simulink model "acc_and_enc"  (R2020a)
settings: Solver=FixedStepDiscrete  StartTime=0.0  StopTime=inf  FixedStep=.001  RelTol=1e-3  EnableMultiTasking=on
undefined symbols (not defined in the file): CAN_Device, Vector
libraries: sldrtlib x2
settings Model: SimulationMode=external  ExtModeTrigDuration=120000  ExtModeLogAll=off  Creator=quinteha  LastModifiedBy=rhyme
settings DataIOCC: LimitDataPoints=on  SaveFormat=Array  ReturnWorkspaceOutputs=off
settings OptimizationCC: ExpressionDepthLimit=2147483647
settings DebuggingCC: UnderspecifiedInitializationDetection=Classic  MergeDetectMultiDrivingBlocksExec=none  SolverPrmCheckMsg=warning  FcnCallInpInsideContextMsg=warning  StateNameClashWarn=warning  SFUnexpectedBacktrackingDiag=warning  SFNoUnconditionalDefaultTransitionDiag=warning  SFExecutionAtInitializationDiag=none  ArithmeticOperatorsInVariantConditions=warning
settings ModelReferenceCC: PropagateSignalLabelsOutOfModel=off
settings SFSimCC: SimUseLocalCustomCode=off  CustomCodeUndefinedFunction=UseInterfaceOnly
settings RTWCC: Description=Simulink Desktop Real-Time  SystemTargetFile=sldrt.tlc  TemplateMakefile=sldrt.tmf  RTWUseLocalCustomCode=off  RTWCompilerOptimization=on
settings CodeAppCC: MaxIdLength=95  StateflowObjectComments=on
settings SimulinkDesktopRealTimeCC: TargetPreCompLibLocation=C:\Program Files\MATLAB\R2020a\toolbox\sldrt\lib\win64  TargetLangStandard=C89/C90 (ANSI)  SupportVariableSizeSignals=off
settings ConfigComp: CovMetricSettings=dw  CovHtmlReporting=on  CovSaveCumulativeToWorkspaceVar=on  CovSaveSingleToWorkspaceVar=on  CovExternalEMLEnable=off  CovSFcnEnable=off

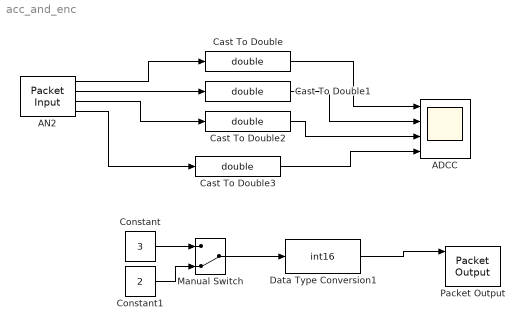
== system acc_and_enc ==
  ADCC : Scope  NumInputPorts=4
  AN2 : sldrtlib/Packet Input  SampleTime=.001  MaxMissedTicks=10  ShowMissedTicks=off  YieldWhenWaiting=off  DrvName=Vector/CAN_Device  DrvAddress=1  DrvOptions=[0 0 0 0 1000]  PacketSize=8  DataTypes={'int16','int16','int16','int16'}  ShowReady=off  ShowError=off  PacketID=2048e0 + (hex2dec('20'))  ByteOrder=1  ShowTimestamp=off
      settings: AttributesFormatString=Vector\nCAN Device [1]
  Cast To Double{,1..3} (4 alike) : DataTypeConversion  OutDataTypeStr=double
  Constant : Constant  Value=3
  Constant1 : Constant  Value=2
  Data Type Conversion1 : DataTypeConversion  OutDataTypeStr=int16
  Manual Switch : ManualSwitch  CurrentSetting=0
  Packet Output : sldrtlib/Packet Output  SampleTime=0.001  MaxMissedTicks=10  ShowMissedTicks=off  YieldWhenWaiting=off  DrvName=Vector/CAN_Device  DrvAddress=1  DrvOptions=[0 0 0 0 1000]  PacketSize=8  DataTypes={'int16','int16','int16','int16'}  ShowReady=off  ShowError=off  PacketID=2048e0 + (hex2dec('80'))  ByteOrder=1  InitialValue=[]  FinalValue=[]
      settings: AttributesFormatString=Vector\nCAN Device [1]
  wires:
  Data Type Conversion1/1 -> Packet Output/1
  Manual Switch/1 -> Data Type Conversion1/1
  Constant/1 -> Manual Switch/1
  Constant1/1 -> Manual Switch/2
  AN2/1 -> Cast To Double/1
  Cast To Double/1 -> ADCC/1
  Cast To Double1/1 -> ADCC/2
  AN2/2 -> Cast To Double1/1
  AN2/3 -> Cast To Double2/1
  Cast To Double2/1 -> ADCC/3
  AN2/4 -> Cast To Double3/1
  Cast To Double3/1 -> ADCC/4
